simulink library "nmc"  (R2015b)
settings: Solver=ode45  SolverMode=SingleTasking  StartTime=0.0  StopTime=10.0  RelTol=1e-3
undefined symbols (not defined in the file): AFOFS_DIM, alphaFmGas, alphaFmGlu, alphaFmHam, alphaFmSol, alphaFmVas, alphaLceHam, alphaLceHfl, alphaLceTa, alphaLceTa1, Amp, amp_var, c, c_jointstop, CPG, D1G_HAT, DeltaThRef, eref, FmaxGAS, FmaxGLU, FmaxHAM, FmaxHFL, FmaxSOL, FmaxTA, FmaxVAS, freq, freq_var, GainDeltaTheta, GainGAS, GainGLU, GainHAM, GainHAMHFL, GainHFL, GainKneOverExt, GainSOL, GainSOLTA, GainTA, GainVAS, K, K_swing, KneePh23Offset, LceOffsetHAM, LceOffsetHFL, LceOffsetTA, left, LongDelay, loptGAS, loptGLU, loptHAM, loptHFL, loptSOL, loptTA, loptVAS, Lphi230, lslackGAS, lslackGLU, lslackHAM, lslackHFL, lslackSOL, lslackTA ... (+66)
libraries: nmc x94, simulink x29, simulink_extras x17
(part 1 of 5)
settings Model: Creator=efx  LastModifiedBy=efx
settings DataIOCC: SaveFormat=Array
settings OptimizationCC: BlockReduction=off  BooleanDataType=off
settings DebuggingCC: SaveWithParameterizedLinksMsg=none  UnderspecifiedInitializationDetection=Classic  MergeDetectMultiDrivingBlocksExec=none  SignalResolutionControl=TryResolveAllWithWarning  StrictBusMsg=Warning
settings HardwareCC: ProdBitPerPointer=32  ProdLargestAtomicFloat=None  ProdIntDivRoundTo=Undefined  ProdEndianess=Unspecified  ProdWordSize=32  ProdHWDeviceType=32-bit Generic  TargetUnknown=on
settings GRTTargetCC: GeneratePreprocessorConditionals=Disable all
settings ConfigComp: CovModelRefEnable=Off  CovSFcnEnable=off

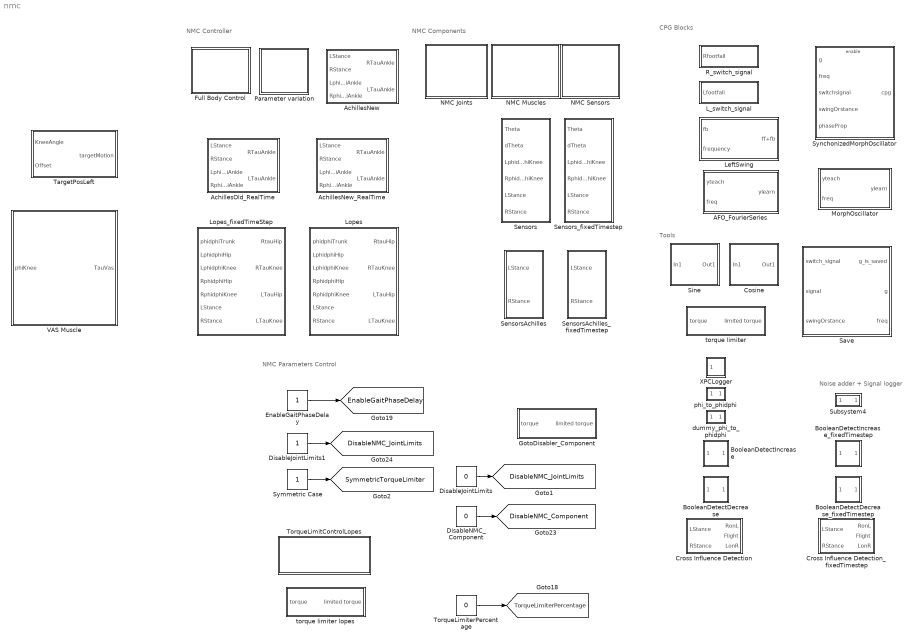
== system nmc ==
  note: Noise adder + Signal logger
  note: NMC Components
  note: Tools
  note: CPG Blocks
  note: NMC Controller
  note: NMC Parameters Control
  AFO_FourierSeries : Subsystem
  AchillesNew : Subsystem
  AchillesNew_RealTime : Subsystem
  AchillesOld_RealTime : Subsystem
  BooleanDetectDecrease : Subsystem
  BooleanDetectDecrease_fixedTimestep : Subsystem
  BooleanDetectIncrease : Subsystem
  BooleanDetectIncrease_fixedTimestep : Subsystem
  Cosine : Subsystem
  Cross Influence Detection : Subsystem
  Cross Influence Detection_fixedTimestep : Subsystem
  DisableJointLimits : Constant  Value=0
  DisableJointLimits1 : Constant
  DisableNMC_Component : Constant  Value=0
  EnableGaitPhaseDelay : Constant
  Full Body Control : Subsystem
  GotoDisabler_Component : Subsystem  mask{GotoTag=DisableNMC_Component}
      mask prompts: GotoTag "Simulink:blkprm_prompts:FromGotoTag"
      mask TypeOptions GotoTag: From/GotoTag
  L_switch_signal : Subsystem
  LeftSwing : Subsystem  InitFcn=CPG.initCurrent();  StopFcn=CPG.saveCurrent();  mask{SaveName=NominalShape1}
      mask prompts: SaveName "Signal nominal shape name"
      mask init:
      | evalin('base','CPG.initCPG();');
      settings: CopyFcn=CPG.initCPG_automaticName();
  Lopes : Subsystem
  Lopes_fixedTimeStep : Subsystem
  MorphOscillator : Subsystem
  NMC Joints : Subsystem
  NMC Muscles : Subsystem
  NMC Sensors : Subsystem
  Parameter variation : Subsystem
  R_switch_signal : Subsystem
  Save : Subsystem
  Sensors : Subsystem
  SensorsAchilles : Subsystem
  SensorsAchilles_fixedTimestep : Subsystem
  Sensors_fixedTimestep : Subsystem
  Sine : Subsystem
  Subsystem4 : Subsystem  mask{GotoTag=LEFT_GLU_FORCE, GotoTag2=LEFT_GLU_FORCE_LOG, GotoTag3=LEFT_GLU_FORCE_NOISE_LOG}
      mask prompts: GotoTag "noise input goto"; GotoTag2 "Goto Logger name"; GotoTag3 "Simulink:blkprm_prompts:GotoTag"
      mask TypeOptions GotoTag: From2/GotoTag
      mask TypeOptions GotoTag2: Goto/GotoTag
      mask TypeOptions GotoTag3: Goto1/GotoTag
  Symmetric Case : Constant
  SynchonizedMorphOscillator : Subsystem
  TargetPosLeft : Subsystem
  TorqueLimitControlLopes : Subsystem
  TorqueLimiterPercentage : Constant  Value=0
  VAS Muscle : Subsystem
  XPCLogger : Subsystem
  dummy_phi_to_phidphi : Subsystem
  phi_to_phidphi : Subsystem
  torque limiter : Subsystem  mask{GotoTag=TorqueLimiterPercentage}
      mask prompts: GotoTag "Simulink:blkprm_prompts:FromGotoTag"
      mask TypeOptions GotoTag: From/GotoTag
  torque limiter lopes : Subsystem  mask{TorqueLimiterPercentage=TorqueLimiterPercentage, EnableTorqueLimiter=EnableTorqueLimiter}
      mask prompts: TorqueLimiterPercentage "Simulink:blkprm_prompts:FromGotoTag"; EnableTorqueLimiter "Simulink:blkprm_prompts:FromGotoTag"
      mask TypeOptions TorqueLimiterPercentage: From/GotoTag
      mask TypeOptions EnableTorqueLimiter: From1/GotoTag
  tag scope: DisableNMC_Component=global, DisableNMC_JointLimits=global, EnableGaitPhaseDelay=global, SymmetricTorqueLimiter=global, TorqueLimiterPercentage=global
  wires:
  TorqueLimiterPercentage/1 -> [TorqueLimiterPercentage]
  DisableNMC_Component/1 -> [DisableNMC_Component]
  DisableJointLimits/1 -> [DisableNMC_JointLimits]
  DisableJointLimits1/1 -> [DisableNMC_JointLimits]
  Symmetric Case/1 -> [SymmetricTorqueLimiter]
  EnableGaitPhaseDelay/1 -> [EnableGaitPhaseDelay]

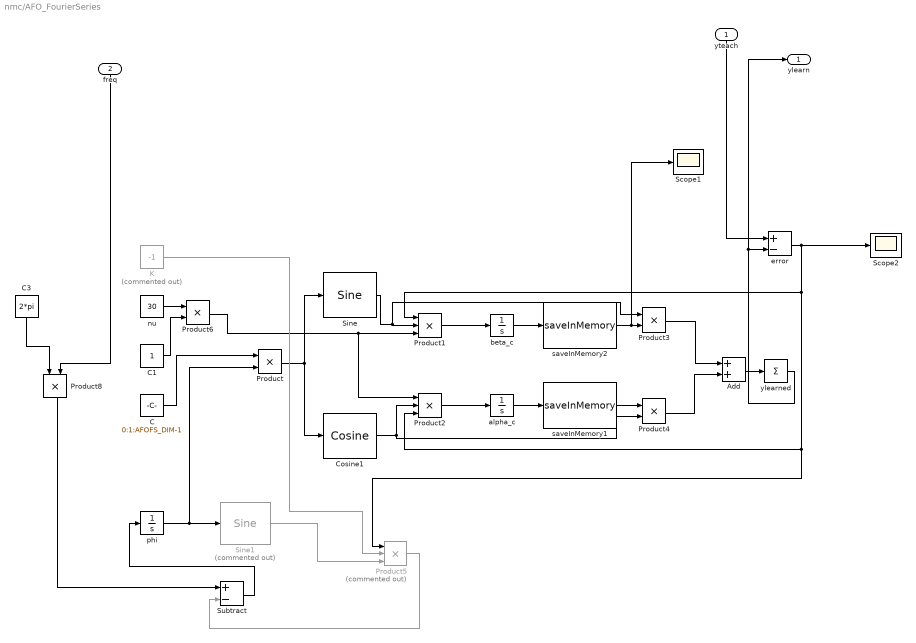
== system nmc/AFO_FourierSeries ==
  yteach : Inport
  freq : Inport  Port=2
  Add : Sum
  C : Constant  Value=0:1:AFOFS_DIM-1
  C1 : Constant
  C3 : Constant  Value=2*pi
  Cosine1 : nmc/Cosine
  K : Constant  Commented=on  Value=-1
  Product{,3..4,6,8} (5 alike) : Product
  Product1 : Product  Inputs=3
  Product2 : Product  Inputs=3
  Product5 : Product  Commented=on  Inputs=3
  Scope1 : Scope
  Scope2 : Scope
  Sine : nmc/Sine
  Sine1 : simulink/Lookup Tables/Sine  Commented=on  Formula=sin(2*pi*u)  NumDataPoints=(2^5)+1  OutputWordLength=16  InternalRulePriority=Speed
  Subtract : Sum  Inputs=+-
  alpha_c : Integrator
  beta_c : Integrator
  error : Sum  Inputs=+-
  nu : Constant  Value=30
  phi : Integrator
  saveInMemory1 : nmc/saveInMemory
  saveInMemory2 : nmc/saveInMemory
  ylearned : Sum  Inputs=+
  ylearn : Outport
  wires:
  saveInMemory2/1 -> Product3/2, Scope1/1
  saveInMemory1/1 -> Product4/1
  yteach/1 -> error/1
  Subtract/1 -> phi/1
  Product6/1 -> Product2/1, Product1/3
  Sine1/1 -> Product5/3
  nu/1 -> Product6/1
  C1/1 -> Product6/2
  Product/1 -> Cosine1/1, Sine/1
  Product1/1 -> beta_c/1
  Product2/1 -> alpha_c/1
  beta_c/1 -> saveInMemory2/1
  alpha_c/1 -> saveInMemory1/1
  Product3/1 -> Add/1
  Product4/1 -> Add/2
  Add/1 -> ylearned/1
  ylearned/1 -> ylearn/1, error/2
  K/1 -> Product5/2
  error/1 -> Product1/1, Product2/3, Product5/1, Scope2/1
  Product5/1 -> Subtract/2
  Product8/1 -> Subtract/1
  phi/1 -> Sine1/1, Product/2
  C/1 -> Product/1
  Sine/1 -> Product1/2, Product3/1
  Cosine1/1 -> Product2/2, Product4/2
  freq/1 -> Product8/2
  C3/1 -> Product8/1

== system nmc/AchillesNew ==
  LStance : Inport
  RStance : Inport  Port=2
  LphidphiAnkle : Inport  Port=3
  RphidphiAnkle : Inport  Port=4
  Left Side : Subsystem
  Right Side : Subsystem
  SensorsAchilles : nmc/SensorsAchilles
  RTauAnkle : Outport
  LTauAnkle : Outport  Port=2
  wires:
  [RTauAnkle] -> RTauAnkle/1
  [LTauAnkle] -> LTauAnkle/1
  Left Side/1(LTauAnkle) -> [LTauAnkle]
  Right Side/1(RTauAnkle) -> [RTauAnkle]
  [RphidphiAnkle] -> Right Side/1(RphidphiAnkle)
  [LphidphiAnkle] -> Left Side/1(LphidphiAnkle)
  RphidphiAnkle/1 -> [RphidphiAnkle]
  LphidphiAnkle/1 -> [LphidphiAnkle]
  [LStance] -> SensorsAchilles/1
  [RStance] -> SensorsAchilles/2
  LStance/1 -> [LStance]
  RStance/1 -> [RStance]

== system nmc/AchillesNew_RealTime ==
  LStance : Inport
  RStance : Inport  Port=2
  LphidphiAnkle : Inport  Port=3
  RphidphiAnkle : Inport  Port=4
  Left Side : Subsystem
  Right Side : Subsystem
  SensorsAchilles_fixedTimestep : nmc/SensorsAchilles_fixedTimestep
  RTauAnkle : Outport
  LTauAnkle : Outport  Port=2
  wires:
  RStance/1 -> [RStance]
  LStance/1 -> [LStance]
  [RStance] -> SensorsAchilles_fixedTimestep/2
  [LStance] -> SensorsAchilles_fixedTimestep/1
  LphidphiAnkle/1 -> [LphidphiAnkle]
  RphidphiAnkle/1 -> [RphidphiAnkle]
  [LphidphiAnkle] -> Left Side/1(LphidphiAnkle)
  [RphidphiAnkle] -> Right Side/1(RphidphiAnkle)
  Right Side/1(RTauAnkle) -> [RTauAnkle]
  Left Side/1(LTauAnkle) -> [LTauAnkle]
  [LTauAnkle] -> LTauAnkle/1
  [RTauAnkle] -> RTauAnkle/1

== system nmc/AchillesOld_RealTime ==
  LStance : Inport
  RStance : Inport  Port=2
  LphidphiAnkle : Inport  Port=3
  RphidphiAnkle : Inport  Port=4
  Achilles : Subsystem
  SensorsAchilles_fixedTimestep : nmc/SensorsAchilles_fixedTimestep
  RTauAnkle : Outport
  LTauAnkle : Outport  Port=2
  wires:
  [RTauAnkle] -> RTauAnkle/1
  [LTauAnkle] -> LTauAnkle/1
  Achilles/1(Torque) -> [LTauAnkle]
  [LphidphiAnkle] -> Achilles/1(AngleLeft)
  RphidphiAnkle/1 -> [RphidphiAnkle]
  LphidphiAnkle/1 -> [LphidphiAnkle]
  [LStance] -> SensorsAchilles_fixedTimestep/1
  [RStance] -> SensorsAchilles_fixedTimestep/2
  LStance/1 -> [LStance]
  RStance/1 -> [RStance]
  [RphidphiAnkle] -> Achilles/3(AngleRight)
  [LstanceOut] -> Achilles/2(IsStanceLeft)
  [RstanceOut] -> Achilles/4(IsStanceRight)
  Achilles/2(Torque1) -> [RTauAnkle]

== system nmc/BooleanDetectDecrease ==
  In1 : Inport
  Compare To Constant : simulink/Logic and Bit Operations/Compare To Constant  relop===  const=-1  OutDataTypeStr=boolean
  Data Type Conversion : DataTypeConversion
  Memory1 : Memory
  Sum : Sum  Inputs=|+-
  Out1 : Outport
  wires:
  Data Type Conversion/1 -> Out1/1
  In1/1 -> Memory1/1, Sum/1
  Sum/1 -> Compare To Constant/1
  Compare To Constant/1 -> Data Type Conversion/1
  Memory1/1 -> Sum/2

== system nmc/BooleanDetectDecrease_fixedTimestep ==
  In1 : Inport
  Data Type Conversion : DataTypeConversion
  Detect Decrease : simulink/Logic and Bit Operations/Detect Decrease  vinit=0.0  InputProcessing=Inherited  OutDataTypeStr=boolean
  Out1 : Outport
  wires:
  In1/1 -> Detect Decrease/1
  Data Type Conversion/1 -> Out1/1
  Detect Decrease/1 -> Data Type Conversion/1

== system nmc/BooleanDetectIncrease ==
  In1 : Inport
  Compare To Constant : simulink/Logic and Bit Operations/Compare To Constant  relop===  const=1  OutDataTypeStr=boolean
  Data Type Conversion : DataTypeConversion
  Memory1 : Memory
  Sum : Sum  Inputs=|+-
  Out1 : Outport
  wires:
  Data Type Conversion/1 -> Out1/1
  In1/1 -> Memory1/1, Sum/1
  Sum/1 -> Compare To Constant/1
  Compare To Constant/1 -> Data Type Conversion/1
  Memory1/1 -> Sum/2

== system nmc/BooleanDetectIncrease_fixedTimestep ==
  In1 : Inport
  Data Type Conversion : DataTypeConversion
  Detect Increase : simulink/Logic and Bit Operations/Detect Increase  vinit=0  InputProcessing=Inherited  OutDataTypeStr=boolean
  Out1 : Outport
  wires:
  Detect Increase/1 -> Data Type Conversion/1
  In1/1 -> Detect Increase/1
  Data Type Conversion/1 -> Out1/1

== system nmc/Cosine ==
  In1 : Inport
  MATLAB Function1 : MATLAB Function  TreatAsAtomicUnit=on
  Out1 : Outport
  wires:
  In1/1 -> MATLAB Function1/1(t)
  MATLAB Function1/1(y) -> Out1/1

== system nmc/Cross Influence Detection ==
  note: Double Support Cross Influences
  note: right leg is leading
  note: left leg is leading
  LStance : Inport  OutDataTypeStr=double
  RStance : Inport  Port=2  OutDataTypeStr=double
  BooleanDetectDecrease : nmc/BooleanDetectDecrease
  BooleanDetectIncrease : nmc/BooleanDetectIncrease
  BooleanDetectIncrease1 : nmc/BooleanDetectIncrease
  Data Type Conversion1 : DataTypeConversion
  Data Type Conversion2 : DataTypeConversion
  Data Type Conversion3 : DataTypeConversion
  Double Support? : Logic  AllPortsSameDT=off
  Double Support?1 : Logic  AllPortsSameDT=off
  Double Support?4 : Logic  AllPortsSameDT=off
  Flight? : Logic  Operator=NOR  AllPortsSameDT=off
  Memory : Memory
  Memory3 : Memory
  S-R Flip-Flop : simulink_extras/Flip Flops/S-R Flip-Flop  initial_condition=0
  S-R Flip-Flop1 : simulink_extras/Flip Flops/S-R Flip-Flop  initial_condition=0
  Terminator1 : Terminator
  Terminator2 : Terminator
  RonL : Outport  OutDataTypeStr=double
  Flight : Outport  Port=2  OutDataTypeStr=double
  LonR : Outport  Port=3  OutDataTypeStr=double
  wires:
  Double Support?1/1 -> S-R Flip-Flop1/1
  BooleanDetectIncrease1/1 -> Double Support?1/2
  S-R Flip-Flop/2 -> Terminator1/1
  S-R Flip-Flop1/2 -> Terminator2/1
  Memory/1 -> BooleanDetectIncrease1/1
  LStance/1 -> Memory3/1, Double Support?/1, Flight?/1
  BooleanDetectIncrease/1 -> Double Support?4/1
  Double Support?4/1 -> S-R Flip-Flop/1
  Memory3/1 -> BooleanDetectIncrease/1
  RStance/1 -> Memory/1, Double Support?/2, Flight?/2
  Double Support?/1 -> BooleanDetectDecrease/1, Double Support?1/1, Double Support?4/2
  S-R Flip-Flop/1 -> Data Type Conversion2/1
  Flight?/1 -> Data Type Conversion1/1
  S-R Flip-Flop1/1 -> Data Type Conversion3/1
  Data Type Conversion1/1 -> Flight/1
  Data Type Conversion2/1 -> LonR/1
  Data Type Conversion3/1 -> RonL/1
  BooleanDetectDecrease/1 -> S-R Flip-Flop/2, S-R Flip-Flop1/2

== system nmc/Cross Influence Detection_fixedTimestep ==
  note: left leg is leading
  note: right leg is leading
  note: Double Support Cross Influences
  LStance : Inport  OutDataTypeStr=double
  RStance : Inport  Port=2  OutDataTypeStr=double
  BooleanDetectDecrease_fixedTimestep : nmc/BooleanDetectDecrease_fixedTimestep
  BooleanDetectIncrease_fixedTimestep : nmc/BooleanDetectIncrease_fixedTimestep
  BooleanDetectIncrease_fixedTimestep1 : nmc/BooleanDetectIncrease_fixedTimestep
  Data Type Conversion1 : DataTypeConversion
  Data Type Conversion2 : DataTypeConversion
  Data Type Conversion3 : DataTypeConversion
  Double Support? : Logic  AllPortsSameDT=off
  Double Support?1 : Logic  AllPortsSameDT=off
  Double Support?4 : Logic  AllPortsSameDT=off
  Flight? : Logic  Operator=NOR  AllPortsSameDT=off
  Memory : Memory
  Memory3 : Memory
  S-R Flip-Flop : simulink_extras/Flip Flops/S-R Flip-Flop  initial_condition=0
  S-R Flip-Flop1 : simulink_extras/Flip Flops/S-R Flip-Flop  initial_condition=0
  Terminator1 : Terminator
  Terminator2 : Terminator
  RonL : Outport  OutDataTypeStr=double
  Flight : Outport  Port=2  OutDataTypeStr=double
  LonR : Outport  Port=3  OutDataTypeStr=double
  wires:
  BooleanDetectDecrease_fixedTimestep/1 -> S-R Flip-Flop1/2, S-R Flip-Flop/2
  Data Type Conversion3/1 -> RonL/1
  Data Type Conversion2/1 -> LonR/1
  Data Type Conversion1/1 -> Flight/1
  S-R Flip-Flop1/1 -> Data Type Conversion3/1
  Flight?/1 -> Data Type Conversion1/1
  S-R Flip-Flop/1 -> Data Type Conversion2/1
  Double Support?/1 -> Double Support?4/2, BooleanDetectDecrease_fixedTimestep/1, Double Support?1/1
  RStance/1 -> Flight?/2, Double Support?/2, Memory/1
  Memory3/1 -> BooleanDetectIncrease_fixedTimestep/1
  Double Support?4/1 -> S-R Flip-Flop/1
  BooleanDetectIncrease_fixedTimestep/1 -> Double Support?4/1
  LStance/1 -> Flight?/1, Double Support?/1, Memory3/1
  Memory/1 -> BooleanDetectIncrease_fixedTimestep1/1
  S-R Flip-Flop1/2 -> Terminator2/1
  S-R Flip-Flop/2 -> Terminator1/1
  BooleanDetectIncrease_fixedTimestep1/1 -> Double Support?1/2
  Double Support?1/1 -> S-R Flip-Flop1/1

== system nmc/Full Body Control ==
  Left Side : Subsystem
  Right Side : Subsystem
  Sensors : Subsystem

== system nmc/GotoDisabler_Component ==
  torque : Inport
  Product : Product
  limited torque : Outport
  wires:
  [DisableNMC_Component] -> Product/1
  Product/1 -> limited torque/1
  torque/1 -> Product/2

== system nmc/L_switch_signal ==
  Lfootfall : Inport
  Memory : Memory
  Subtract : Sum  Inputs=+-
  tag scope: CPG_leftSwitchSignal=global
  wires:
  Subtract/1 -> [CPG_leftSwitchSignal]
  Lfootfall/1 -> Memory/1, Subtract/1
  Memory/1 -> Subtract/2

== system nmc/LeftSwing ==
  fb : Inport
  frequency : Inport  Port=2
  AlreadySavedInWorkspace : Constant  Value=CPG.Signals.NominalShape1.Enabled
  CPG : Subsystem
  ChooseOutput : Switch  Criteria=u2 > Threshold  Threshold=0.5
  GenerateAndSaveNominalShape : Subsystem
  LeftOrRight : Subsystem
  Logical Operator : Logic  Operator=NOT  Inputs=1  AllPortsSameDT=off  OutDataTypeStr=boolean
  leftOrright : Constant  Value=left
  swingOrstance : Constant  Value=swing
  ff+fb : Outport
  wires:
  LeftOrRight/1(switch_signal) -> GenerateAndSaveNominalShape/1(switch_signal)
  leftOrright/1 -> LeftOrRight/1(side)
  ChooseOutput/1 -> ff+fb/1
  frequency/1 -> CPG/1(freq)
  CPG/1(y) -> ChooseOutput/1
  Logical Operator/1 -> GenerateAndSaveNominalShape/Enable
  swingOrstance/1 -> GenerateAndSaveNominalShape/3(swingOrstance)
  fb/1 -> ChooseOutput/3, GenerateAndSaveNominalShape/2(signal)
  AlreadySavedInWorkspace/1 -> CPG/Enable, ChooseOutput/2, Logical Operator/1

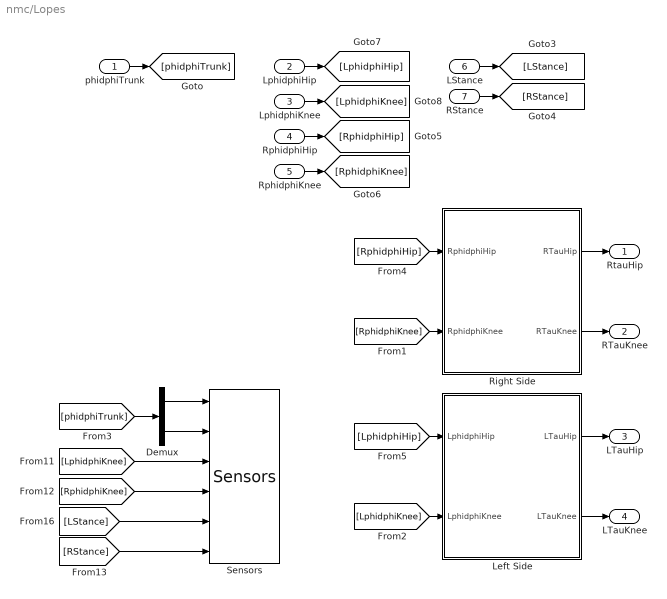
== system nmc/Lopes ==
  phidphiTrunk : Inport
  LphidphiHip : Inport  Port=2
  LphidphiKnee : Inport  Port=3
  RphidphiHip : Inport  Port=4
  RphidphiKnee : Inport  Port=5
  LStance : Inport  Port=6
  RStance : Inport  Port=7
  Demux : Demux  Outputs=2
  Left Side : Subsystem
  Right Side : Subsystem
  Sensors : nmc/Sensors
  RtauHip : Outport
  RTauKnee : Outport  Port=2
  LTauHip : Outport  Port=3
  LTauKnee : Outport  Port=4
  wires:
  RphidphiKnee/1 -> [RphidphiKnee]
  LphidphiHip/1 -> [LphidphiHip]
  LphidphiKnee/1 -> [LphidphiKnee]
  RphidphiHip/1 -> [RphidphiHip]
  RStance/1 -> [RStance]
  LStance/1 -> [LStance]
  phidphiTrunk/1 -> [phidphiTrunk]
  Left Side/2(LTauKnee) -> LTauKnee/1
  Left Side/1(LTauHip) -> LTauHip/1
  Right Side/2(RTauKnee) -> RTauKnee/1
  Right Side/1(RTauHip) -> RtauHip/1
  [LphidphiHip] -> Left Side/1(LphidphiHip)
  [RphidphiHip] -> Right Side/1(RphidphiHip)
  Demux/2 -> Sensors/2
  Demux/1 -> Sensors/1
  [phidphiTrunk] -> Demux/1
  [LphidphiKnee] -> Left Side/2(LphidphiKnee)
  [RphidphiKnee] -> Right Side/2(RphidphiKnee)
  [RStance] -> Sensors/6
  [LStance] -> Sensors/5
  [RphidphiKnee] -> Sensors/4
  [LphidphiKnee] -> Sensors/3

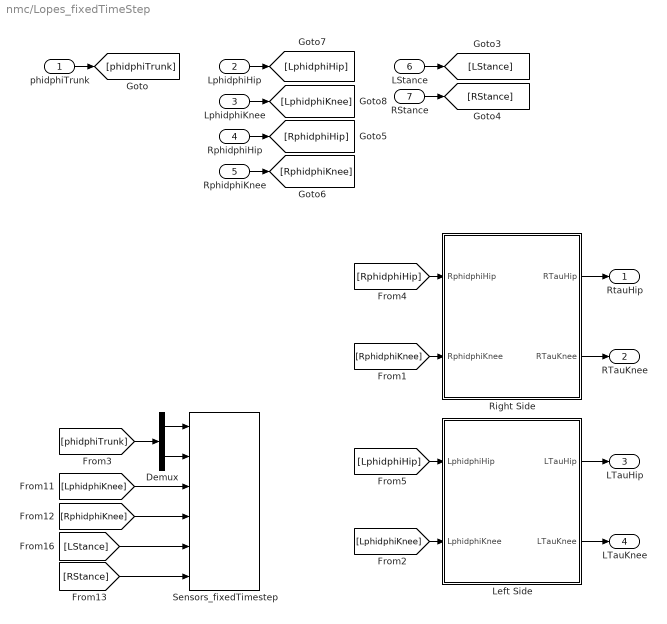
== system nmc/Lopes_fixedTimeStep ==
  phidphiTrunk : Inport
  LphidphiHip : Inport  Port=2
  LphidphiKnee : Inport  Port=3
  RphidphiHip : Inport  Port=4
  RphidphiKnee : Inport  Port=5
  LStance : Inport  Port=6
  RStance : Inport  Port=7
  Demux : Demux  Outputs=2
  Left Side : Subsystem
  Right Side : Subsystem
  Sensors_fixedTimestep : nmc/Sensors_fixedTimestep
  RtauHip : Outport
  RTauKnee : Outport  Port=2
  LTauHip : Outport  Port=3
  LTauKnee : Outport  Port=4
  wires:
  [LphidphiKnee] -> Sensors_fixedTimestep/3
  [RphidphiKnee] -> Sensors_fixedTimestep/4
  [LStance] -> Sensors_fixedTimestep/5
  [RStance] -> Sensors_fixedTimestep/6
  [RphidphiKnee] -> Right Side/2(RphidphiKnee)
  [LphidphiKnee] -> Left Side/2(LphidphiKnee)
  [phidphiTrunk] -> Demux/1
  Demux/1 -> Sensors_fixedTimestep/1
  Demux/2 -> Sensors_fixedTimestep/2
  [RphidphiHip] -> Right Side/1(RphidphiHip)
  [LphidphiHip] -> Left Side/1(LphidphiHip)
  Right Side/1(RTauHip) -> RtauHip/1
  Right Side/2(RTauKnee) -> RTauKnee/1
  Left Side/1(LTauHip) -> LTauHip/1
  Left Side/2(LTauKnee) -> LTauKnee/1
  phidphiTrunk/1 -> [phidphiTrunk]
  LStance/1 -> [LStance]
  RStance/1 -> [RStance]
  RphidphiHip/1 -> [RphidphiHip]
  LphidphiKnee/1 -> [LphidphiKnee]
  LphidphiHip/1 -> [LphidphiHip]
  RphidphiKnee/1 -> [RphidphiKnee]

== system nmc/MorphOscillator ==
  yteach : Inport
  freq : Inport  Port=2
  Digital Clock : DigitalClock  SampleTime=0.001
  MATLAB Function : MATLAB Function  TreatAsAtomicUnit=on
  ylearn : Outport  SampleTime=0.001
  wires:
  freq/1 -> MATLAB Function/2(freq)
  yteach/1 -> MATLAB Function/1(g)
  Digital Clock/1 -> MATLAB Function/3(t)
  MATLAB Function/1(y) -> ylearn/1

== system nmc/NMC Joints ==
  AnkleJoint : Subsystem
  HipJoint : Subsystem
  KneeJoint : Subsystem

== system nmc/NMC Muscles ==
  note: NMC Muscles
  GAS Muscle : Subsystem  mask{VariableName=StimGAS, GASVM=GASL_VM}
      mask prompts: VariableName "Simulink:blkprm_prompts:ToWksVarName"; GASVM "Simulink:blkprm_prompts:GotoTag"
      mask TypeOptions VariableName: StimGAS/VariableName
      mask TypeOptions GASVM: GAS Actuation / GAS_VM/GotoTag
  GLU Muscle : Subsystem  mask{StimGluSide=StimGLUR, GotoTag=GLUR_VM}
      mask prompts: StimGluSide "Simulink:blkprm_prompts:ToWksVarName"; GotoTag "Simulink:blkprm_prompts:GotoTag"
      mask TypeOptions StimGluSide: StimGLU/VariableName
      mask TypeOptions GotoTag: GLU Actuation/GLU_VM /GotoTag
  "HFL Muscle " : Subsystem  mask{VariableName=StimHFL}
      mask prompts: VariableName "Simulink:blkprm_prompts:ToWksVarName"
      mask TypeOptions VariableName: StimHFL/VariableName
  HFL&HAM Muscles : Subsystem  mask{StimHAMSide=StimHAMR, StimHFLSide=StimHFLR, HAMVM=HAMR_VM, HFLVM=HFLR_VM}
      mask prompts: StimHAMSide "Simulink:blkprm_prompts:ToWksVarName"; StimHFLSide "Simulink:blkprm_prompts:ToWksVarName"; HAMVM "Simulink:blkprm_prompts:GotoTag"; HFLVM "Simulink:blkprm_prompts:GotoTag"
      mask TypeOptions StimHAMSide: StimHAM/VariableName
      mask TypeOptions StimHFLSide: StimHFL/VariableName
      mask TypeOptions HAMVM: HAM Actuation / HAM_VM/GotoTag
      mask TypeOptions HFLVM: HFL Actuation/ HFL_VM/GotoTag
  SOL&TA Muscles : Subsystem  mask{VariableName=StimSOL, VariableNameTA=StimTA, SOLVM=SOLL_VM, TAVM=TAL_VM}
      mask prompts: VariableName "Simulink:blkprm_prompts:ToWksVarName"; VariableNameTA "Simulink:blkprm_prompts:ToWksVarName"; SOLVM "Simulink:blkprm_prompts:GotoTag"; TAVM "Simulink:blkprm_prompts:GotoTag"
      mask TypeOptions VariableName: StimSOL/VariableName
      mask TypeOptions VariableNameTA: StimTA/VariableName
      mask TypeOptions SOLVM: SOL Actuation/SOL_VM/GotoTag
      mask TypeOptions TAVM: TA Actuation/TA_VM/GotoTag
  VAS Muscle : Subsystem  mask{VariableName=StimVASR, VASVM=VASR_VM}
      mask prompts: VariableName "Simulink:blkprm_prompts:ToWksVarName"; VASVM "Simulink:blkprm_prompts:GotoTag"
      mask TypeOptions VariableName: StimVAS/VariableName
      mask TypeOptions VASVM: VAS Actuation / VAS_VM/GotoTag

== system nmc/NMC Sensors ==
  FootSensor : Subsystem
  FootSensorSimple : Subsystem
  FootSensor_fixedTimestep : Subsystem
  GeyerUpperBodyOrientation : Subsystem
  KneeSensor : Subsystem
  ThightSensor : Subsystem
  ThightSensorSimulator : Subsystem
  UpperBodyOrientation : Subsystem

== system nmc/Parameter variation ==
  Alpha variation : Subsystem
  Amplitude Variation : Subsystem
  Freq variation : Subsystem

== system nmc/R_switch_signal ==
  Rfootfall : Inport
  Memory : Memory
  Subtract : Sum  Inputs=+-
  tag scope: CPG_rightSwitchSignal=global
  wires:
  Rfootfall/1 -> Subtract/1, Memory/1
  Memory/1 -> Subtract/2
  Subtract/1 -> [CPG_rightSwitchSignal]

== system nmc/Save ==
  switch_signal : Inport
  signal : Inport  Port=2
  "swingOrstance " : Inport  Port=3
  N_record : Constant  Value=N_record
  N_start : Constant  Value=N_start
  save : Stateflow chart  TreatAsAtomicUnit=on
  g_is_saved : Outport
  g : Outport  Port=2
  freq : Outport  Port=3
  wires:
  save/3(saved) -> g_is_saved/1
  "swingOrstance "/1 -> save/5(swingOrstance)
  save/1(g) -> g/1
  N_start/1 -> save/2(N_start)
  save/2(freq) -> freq/1
  signal/1 -> save/4(signal)
  N_record/1 -> save/3(N_record)
  switch_signal/1 -> save/1(switch_signal)

== system nmc/Sensors ==
  Theta : Inport
  dTheta : Inport  Port=2
  LphidphiKnee : Inport  Port=3
  RphidphiKnee : Inport  Port=4
  LStance : Inport  Port=5
  RStance : Inport  Port=6
  Body Pitch loop delay : TransportDelay  DelayTime=ShortDelay
  Body Pitch loop delay. : TransportDelay  DelayTime=ShortDelay
  FootSensor : nmc/NMC Sensors/FootSensor
  KneeSensor : nmc/NMC Sensors/KneeSensor
  ThightSensorSimulator : nmc/NMC Sensors/ThightSensorSimulator
  To Workspace : ToWorkspace  VariableName=L_GRF  SaveFormat=Timeseries  SampleTime=-1
  To Workspace1 : ToWorkspace  VariableName=R_GRF  SaveFormat=Timeseries  SampleTime=-1
  tag scope: LKneeStateOut=global, LdxThighOut=global, LonR=global, LstanceOut=global, RKneeStateOut=global, RdxThighOut=global, RonL=global, RstanceOut=global, ThetaDelayed=global, dThetaDelayed=global
  wires:
  LphidphiKnee/1 -> KneeSensor/1
  RphidphiKnee/1 -> KneeSensor/2
  KneeSensor/1 -> [LKneeStateOut]
  KneeSensor/2 -> [RKneeStateOut]
  FootSensor/1 -> [LstanceOut]
  FootSensor/2 -> [RstanceOut]
  FootSensor/3 -> [LonR]
  FootSensor/4 -> [RonL]
  ThightSensorSimulator/1 -> [LdxThighOut]
  ThightSensorSimulator/2 -> [RdxThighOut]
  [rightGRF_vertical] -> To Workspace1/1
  [leftGRF_vertical] -> To Workspace/1
  [LstanceOut] -> ThightSensorSimulator/1
  [RstanceOut] -> ThightSensorSimulator/2
  RStance/1 -> FootSensor/2
  LStance/1 -> FootSensor/1
  Theta/1 -> Body Pitch loop delay./1
  dTheta/1 -> Body Pitch loop delay/1
  Body Pitch loop delay./1 -> [ThetaDelayed]
  Body Pitch loop delay/1 -> [dThetaDelayed]

== system nmc/SensorsAchilles ==
  LStance : Inport
  RStance : Inport  Port=2
  FootSensor : nmc/NMC Sensors/FootSensor
  tag scope: LonR=global, LstanceOut=global, RonL=global, RstanceOut=global
  wires:
  LStance/1 -> FootSensor/1
  RStance/1 -> FootSensor/2
  FootSensor/4 -> [RonL]
  FootSensor/3 -> [LonR]
  FootSensor/2 -> [RstanceOut]
  FootSensor/1 -> [LstanceOut]

== system nmc/SensorsAchilles_fixedTimestep ==
  LStance : Inport
  RStance : Inport  Port=2
  FootSensor_fixedTimestep : nmc/NMC Sensors/FootSensor_fixedTimestep
  tag scope: LonR=global, LstanceOut=global, RonL=global, RstanceOut=global
  wires:
  FootSensor_fixedTimestep/1 -> [LstanceOut]
  FootSensor_fixedTimestep/2 -> [RstanceOut]
  FootSensor_fixedTimestep/3 -> [LonR]
  FootSensor_fixedTimestep/4 -> [RonL]
  RStance/1 -> FootSensor_fixedTimestep/2
  LStance/1 -> FootSensor_fixedTimestep/1

== system nmc/Sensors_fixedTimestep ==
  Theta : Inport
  dTheta : Inport  Port=2
  LphidphiKnee : Inport  Port=3
  RphidphiKnee : Inport  Port=4
  LStance : Inport  Port=5
  RStance : Inport  Port=6
  Body Pitch loop delay : TransportDelay  DelayTime=ShortDelay
  Body Pitch loop delay. : TransportDelay  DelayTime=ShortDelay
  FootSensor_fixedTimestep : nmc/NMC Sensors/FootSensor_fixedTimestep
  KneeSensor : nmc/NMC Sensors/KneeSensor
  ThightSensorSimulator : nmc/NMC Sensors/ThightSensorSimulator
  To Workspace : ToWorkspace  VariableName=L_GRF  SaveFormat=Timeseries  SampleTime=-1
  To Workspace1 : ToWorkspace  VariableName=R_GRF  SaveFormat=Timeseries  SampleTime=-1
  tag scope: LKneeStateOut=global, LdxThighOut=global, LonR=global, LstanceOut=global, RKneeStateOut=global, RdxThighOut=global, RonL=global, RstanceOut=global, ThetaDelayed=global, dThetaDelayed=global
  wires:
  Body Pitch loop delay/1 -> [dThetaDelayed]
  Body Pitch loop delay./1 -> [ThetaDelayed]
  dTheta/1 -> Body Pitch loop delay/1
  Theta/1 -> Body Pitch loop delay./1
  LStance/1 -> FootSensor_fixedTimestep/1
  RStance/1 -> FootSensor_fixedTimestep/2
  [RstanceOut] -> ThightSensorSimulator/2
  [LstanceOut] -> ThightSensorSimulator/1
  [leftGRF_vertical] -> To Workspace/1
  [rightGRF_vertical] -> To Workspace1/1
  ThightSensorSimulator/2 -> [RdxThighOut]
  ThightSensorSimulator/1 -> [LdxThighOut]
  FootSensor_fixedTimestep/4 -> [RonL]
  FootSensor_fixedTimestep/3 -> [LonR]
  FootSensor_fixedTimestep/2 -> [RstanceOut]
  FootSensor_fixedTimestep/1 -> [LstanceOut]
  KneeSensor/2 -> [RKneeStateOut]
  KneeSensor/1 -> [LKneeStateOut]
  RphidphiKnee/1 -> KneeSensor/2
  LphidphiKnee/1 -> KneeSensor/1

== system nmc/Sine ==
  In1 : Inport
  MATLAB Function1 : MATLAB Function  TreatAsAtomicUnit=on
  Out1 : Outport
  wires:
  MATLAB Function1/1(y) -> Out1/1
  In1/1 -> MATLAB Function1/1(t)

== system nmc/Subsystem4 ==
  In1 : Inport
  Constant : Constant  Value=0
  Sum : Sum  Inputs=|++
  Switch : Switch  Criteria=u2 > Threshold
  Out1 : Outport
  tag scope: LEFT_GLU_FORCE_LOG=global, LEFT_GLU_FORCE_NOISE_LOG=global
  wires:
  In1/1 -> Sum/2, [LEFT_GLU_FORCE_LOG]
  [LEFT_GLU_FORCE] -> Sum/1
  Sum/1 -> Switch/1, Switch/2
  Constant/1 -> Switch/3
  Switch/1 -> [LEFT_GLU_FORCE_NOISE_LOG], Out1/1

== system nmc/SynchonizedMorphOscillator ==
  g : Inport
  freq : Inport  Port=2
  switchsignal : Inport  Port=3
  swingOrstance : Inport  Port=4
  phaseProp : Inport  Port=5
  Enable : EnablePort
  ConstantCPG : Subsystem
  Logical Operator : Logic  Operator=NOT  AllPortsSameDT=off  OutDataTypeStr=boolean
  Memory : Memory
  Memory1 : Memory
  Memory2 : Memory
  MorphingOscillator : Subsystem
  State Transition Table : State Transition Table  TreatAsAtomicUnit=on
  Switch : Switch  Criteria=u2 > Threshold
  enable cpg : Subsystem
  cpg : Outport
  wires:
  MorphingOscillator/2(tetha_out) -> Memory/1
  swingOrstance/1 -> MorphingOscillator/4(swingOrstance), State Transition Table/2(swingOrstance)
  freq/1 -> MorphingOscillator/2(freq)
  g/1 -> MorphingOscillator/1(g)
  State Transition Table/1(actif) -> Logical Operator/1, enable cpg/Enable, Switch/2
  State Transition Table/2(cpg_cnst) -> ConstantCPG/1(cpg_cnst_value)
  Logical Operator/1 -> ConstantCPG/Enable
  ConstantCPG/1(cpg_value) -> Switch/3
  Switch/1 -> cpg/1
  switchsignal/1 -> MorphingOscillator/3(switchsignal), Memory2/1
  Memory1/1 -> State Transition Table/3(cpg)
  Memory/1 -> State Transition Table/4(tetha)
  MorphingOscillator/1(cpg) -> Memory1/1, enable cpg/1(cpg_on)
  enable cpg/1(cpg) -> Switch/1
  Memory2/1 -> State Transition Table/1(switchsignal)
  phaseProp/1 -> State Transition Table/5(phaseProp)

== system nmc/TargetPosLeft ==
  KneeAngle : Inport
  Offset : Inport  Port=2
  Add : Sum  Inputs=-+
  Add1 : Sum
  Constant : Constant  Value=0
  Constant1 : Constant  Value=pi
  Demux4 : Demux  Outputs=2
  Gain : Gain  Gain=0.5
  Memory : Memory  X0=Lphi230
  Mux1 : Mux  Inputs=3
  Terminator : Terminator
  targetMotion : Outport
  wires:
  KneeAngle/1 -> Memory/1
  Mux1/1 -> targetMotion/1
  Demux4/2 -> Terminator/1
  Constant/1 -> Mux1/3, Mux1/2
  Add/1 -> Gain/1
  Demux4/1 -> Add/2
  Constant1/1 -> Add/1
  Gain/1 -> Add1/2
  Add1/1 -> Mux1/1
  Offset/1 -> Add1/1
  Memory/1 -> Demux4/1

== system nmc/TorqueLimitControlLopes ==
  Constant6 : Constant
  Subtract : Sum  Inputs=-+
  tag scope: EnableAssymmetricTorqueLimiter=global, EnableSymmetricTorqueLimiter=global
  wires:
  [SymmetricTorqueLimiter] -> Subtract/1, [EnableSymmetricTorqueLimiter]
  Subtract/1 -> [EnableAssymmetricTorqueLimiter]
  Constant6/1 -> Subtract/2

== system nmc/VAS Muscle ==
  note: VAS Control
  note: VAS Muscle
  note: VAS Control
  phiKnee : Inport
  "ANMC STIM " : Concatenate  NumInputs=1
  Gain : Gain  Gain=GainVAS
  LOG_TauVas : Concatenate  NumInputs=1
  Saturation17 : Saturate  UpperLimit=1  LowerLimit=0.01  ZeroCross=off
  Stimulation Bias : Constant  Value=PreStimVAS
  Sum2 : Sum  Inputs=|++  SaturateOnIntegerOverflow=on  InputSameDT=on  OutDataTypeStr=Inherit: Same as first input
  "VAS Actuation " : Subsystem
  TauVas : Outport
  wires:
  LOG_TauVas/1 -> TauVas/1
  "ANMC STIM "/1 -> "VAS Actuation "/2(StimVas)
  "VAS Actuation "/1(TauVas) -> LOG_TauVas/1
  phiKnee/1 -> "VAS Actuation "/1(phiKnee)
  "VAS Actuation "/2(FmVas) -> Gain/1
  Gain/1 -> Sum2/2
  Stimulation Bias/1 -> Sum2/1
  Sum2/1 -> Saturation17/1
  Saturation17/1 -> "ANMC STIM "/1

== system nmc/XPCLogger ==
  In1 : Inport
  Terminator5 : Terminator
  wires:
  In1/1 -> Terminator5/1

== system nmc/dummy_phi_to_phidphi ==
  phi : Inport
  Constant : Constant  Value=0
  Mux : Mux  Inputs=2
  phi_dummydphi : Outport
  wires:
  Mux/1 -> phi_dummydphi/1
  phi/1 -> Mux/2
  Constant/1 -> Mux/1

== system nmc/phi_to_phidphi ==
  phi : Inport
  Derivative : Derivative
  LOG_dPHI : Concatenate  NumInputs=1
  Mux : Mux  Inputs=2
  phidphi : Outport
  wires:
  phi/1 -> Mux/1, Derivative/1
  Mux/1 -> phidphi/1
  Derivative/1 -> LOG_dPHI/1
  LOG_dPHI/1 -> Mux/2

== system nmc/torque limiter ==
  torque : Inport
  Gain : Gain  Gain=0.01
  Gain1 : Gain  Gain=-1
  Product : Product
  Saturation : Saturate  UpperLimit=2  LowerLimit=0
  limited torque : Outport
  wires:
  Gain/1 -> Saturation/1
  [TorqueLimiterPercentage] -> Gain/1
  Product/1 -> limited torque/1
  torque/1 -> Product/2
  Gain1/1 -> Product/1
  Saturation/1 -> Gain1/1

== system nmc/torque limiter lopes ==
  torque : Inport
  Gain1 : Gain  Gain=0.01
  Product1 : Product
  Switch : Switch  Criteria=u2 > Threshold
  limited torque : Outport
  wires:
  Gain1/1 -> Product1/1
  [TorqueLimiterPercentage] -> Gain1/1
  torque/1 -> Product1/2, [NonLimitedOutput]
  [EnableTorqueLimiter] -> Switch/2
  Switch/1 -> limited torque/1
  Product1/1 -> [LimitedOutput]
  [LimitedOutput] -> Switch/1
  [NonLimitedOutput] -> Switch/3

== system nmc/AchillesNew/Left Side ==
  LphidphiAnkle : Inport
  AnkleJoint : nmc/NMC Joints/AnkleJoint
  SOL&TA Muscles : nmc/NMC Muscles/SOL&TA Muscles  VariableName=StimSOLL  VariableNameTA=StimTAL  SOLVM=SOLL_VM  TAVM=TAL_VM
  Selector7 : Selector  InputPortWidth=2  IndexOptions=Index vector (dialog)  Indices=[1 ]  OutputSizes=1
  Vector ConcatenateAnkle : Concatenate
  LTauAnkle : Outport
  wires:
  [LstanceOut] -> SOL&TA Muscles/2
  Selector7/1 -> SOL&TA Muscles/1
  [LTauAnkle] -> LTauAnkle/1
  LphidphiAnkle/1 -> [LphidphiAnkle]
  AnkleJoint/1 -> [LTauAnkle]
  [LphidphiAnkle] -> Selector7/1
  [LphidphiAnkle] -> AnkleJoint/1
  SOL&TA Muscles/1 -> Vector ConcatenateAnkle/1
  Vector ConcatenateAnkle/1 -> AnkleJoint/2
  SOL&TA Muscles/2 -> Vector ConcatenateAnkle/2

== system nmc/AchillesNew/Right Side ==
  RphidphiAnkle : Inport
  AnkleJoint : nmc/NMC Joints/AnkleJoint
  SOL&TA Muscles : nmc/NMC Muscles/SOL&TA Muscles  VariableName=StimSOLR  VariableNameTA=StimTAR  SOLVM=SOLL_VM  TAVM=TAL_VM
  Selector7 : Selector  InputPortWidth=2  IndexOptions=Index vector (dialog)  Indices=[1 ]  OutputSizes=1
  Vector ConcatenateAnkle : Concatenate
  RTauAnkle : Outport
  wires:
  [RTauAnkle] -> RTauAnkle/1
  RphidphiAnkle/1 -> [RphidphiAnkle]
  AnkleJoint/1 -> [RTauAnkle]
  [RstanceOut] -> SOL&TA Muscles/2
  [RphidphiAnkle] -> Selector7/1
  [RphidphiAnkle] -> AnkleJoint/1
  SOL&TA Muscles/1 -> Vector ConcatenateAnkle/1
  Vector ConcatenateAnkle/1 -> AnkleJoint/2
  Selector7/1 -> SOL&TA Muscles/1
  SOL&TA Muscles/2 -> Vector ConcatenateAnkle/2

== system nmc/AchillesNew_RealTime/Left Side ==
  LphidphiAnkle : Inport
  AnkleJoint : nmc/NMC Joints/AnkleJoint
  SOL&TA Muscles : nmc/NMC Muscles/SOL&TA Muscles  VariableName=StimSOLL  VariableNameTA=StimTAL  SOLVM=SOLL_VM  TAVM=TAL_VM
  Selector7 : Selector  InputPortWidth=2  IndexOptions=Index vector (dialog)  Indices=[1 ]  OutputSizes=1
  Vector ConcatenateAnkle : Concatenate
  LTauAnkle : Outport
  wires:
  SOL&TA Muscles/2 -> Vector ConcatenateAnkle/2
  Vector ConcatenateAnkle/1 -> AnkleJoint/2
  SOL&TA Muscles/1 -> Vector ConcatenateAnkle/1
  [LphidphiAnkle] -> AnkleJoint/1
  [LphidphiAnkle] -> Selector7/1
  AnkleJoint/1 -> [LTauAnkle]
  LphidphiAnkle/1 -> [LphidphiAnkle]
  [LTauAnkle] -> LTauAnkle/1
  Selector7/1 -> SOL&TA Muscles/1
  [LstanceOut] -> SOL&TA Muscles/2

== system nmc/AchillesNew_RealTime/Right Side ==
  RphidphiAnkle : Inport
  AnkleJoint : nmc/NMC Joints/AnkleJoint
  SOL&TA Muscles : nmc/NMC Muscles/SOL&TA Muscles  VariableName=StimSOLR  VariableNameTA=StimTAR  SOLVM=SOLL_VM  TAVM=TAL_VM
  Selector7 : Selector  InputPortWidth=2  IndexOptions=Index vector (dialog)  Indices=[1 ]  OutputSizes=1
  Vector ConcatenateAnkle : Concatenate
  RTauAnkle : Outport
  wires:
  SOL&TA Muscles/2 -> Vector ConcatenateAnkle/2
  Selector7/1 -> SOL&TA Muscles/1
  Vector ConcatenateAnkle/1 -> AnkleJoint/2
  SOL&TA Muscles/1 -> Vector ConcatenateAnkle/1
  [RphidphiAnkle] -> AnkleJoint/1
  [RphidphiAnkle] -> Selector7/1
  [RstanceOut] -> SOL&TA Muscles/2
  AnkleJoint/1 -> [RTauAnkle]
  RphidphiAnkle/1 -> [RphidphiAnkle]
  [RTauAnkle] -> RTauAnkle/1

== system nmc/AchillesOld_RealTime/Achilles ==
  AngleLeft : Inport
  IsStanceLeft : Inport  Port=2
  AngleRight : Inport  Port=3
  IsStanceRight : Inport  Port=4
  Add1 : Sum
  Add2 : Sum
  NMC_input_LeftAngle : Concatenate  NumInputs=1
  NMC_input_LeftStance : Concatenate  NumInputs=1
  NMC_input_RightAngle : Concatenate  NumInputs=1
  NMC_input_RightStance : Concatenate  NumInputs=1
  SOL&TA muscles left1 : nmc/NMC Muscles/SOL&TA Muscles  VariableName=StimSOLL  VariableNameTA=StimTAL  SOLVM=SOLL_VM  TAVM=TAL_VM
  SOL&TA muscles right : nmc/NMC Muscles/SOL&TA Muscles  VariableName=StimSOLR  VariableNameTA=StimTALR  SOLVM=SOLL_VM  TAVM=TAL_VM
  Torque : Outport
  Torque1 : Outport  Port=2
  wires:
  AngleLeft/1 -> NMC_input_LeftAngle/1
  NMC_input_LeftStance/1 -> SOL&TA muscles left1/2
  SOL&TA muscles left1/1 -> Add1/1
  SOL&TA muscles left1/2 -> Add1/2
  IsStanceLeft/1 -> NMC_input_LeftStance/1
  NMC_input_LeftAngle/1 -> SOL&TA muscles left1/1
  AngleRight/1 -> NMC_input_RightAngle/1
  NMC_input_RightStance/1 -> SOL&TA muscles right/2
  SOL&TA muscles right/1 -> Add2/1
  SOL&TA muscles right/2 -> Add2/2
  IsStanceRight/1 -> NMC_input_RightStance/1
  NMC_input_RightAngle/1 -> SOL&TA muscles right/1
  Add1/1 -> Torque/1
  Add2/1 -> Torque1/1

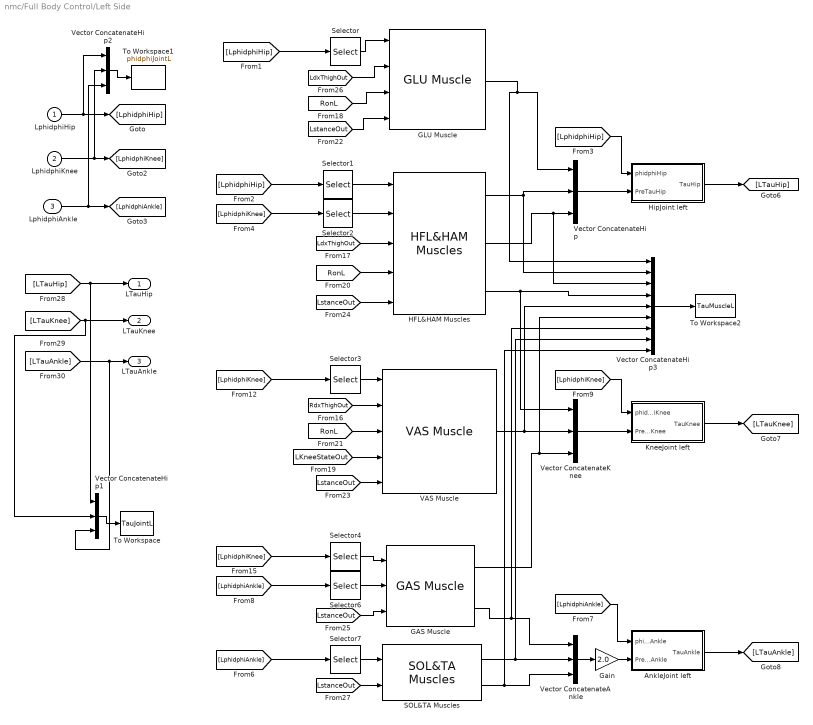
== system nmc/Full Body Control/Left Side ==
  LphidphiHip : Inport
  LphidphiKnee : Inport  Port=2
  LphidphiAnkle : Inport  Port=3
  AnkleJoint left : Subsystem
  GAS Muscle : nmc/NMC Muscles/GAS Muscle  VariableName=StimGASL  GASVM=GASL_VM
  GLU Muscle : nmc/NMC Muscles/GLU Muscle  StimGluSide=StimGLU1  GotoTag=GLUR_VM
  Gain : Gain  Gain=2.0
  HFL&HAM Muscles : nmc/NMC Muscles/HFL&HAM Muscles  StimHAMSide=StimHAM  StimHFLSide=StimHFL  HAMVM=HAMR_VM  HFLVM=HFLR_VM
  HipJoint left : Subsystem
  KneeJoint left : Subsystem
  SOL&TA Muscles : nmc/NMC Muscles/SOL&TA Muscles  VariableName=StimSOLL  VariableNameTA=StimTAL  SOLVM=SOLL_VM  TAVM=TAL_VM
  Selector{,1..4,6..7} (7 alike) : Selector  InputPortWidth=2  IndexOptions=Index vector (dialog)  Indices=[1 ]  OutputSizes=1
  To Workspace : ToWorkspace  VariableName=TauJointL  SaveFormat=Timeseries  SampleTime=-1
  To Workspace1 : ToWorkspace  VariableName=phidphiJointL  SaveFormat=Timeseries  SampleTime=-1
  To Workspace2 : ToWorkspace  VariableName=TauMuscleL  SaveFormat=Timeseries  SampleTime=-1
  VAS Muscle : nmc/NMC Muscles/VAS Muscle  VariableName=StimVAS  VASVM=VASR_VM
  Vector ConcatenateAnkle : Concatenate  NumInputs=3
  Vector ConcatenateHip : Concatenate  NumInputs=3
  Vector ConcatenateHip1 : Concatenate  NumInputs=3
  Vector ConcatenateHip2 : Concatenate  NumInputs=3
  Vector ConcatenateHip3 : Concatenate  NumInputs=9
  Vector ConcatenateKnee : Concatenate  NumInputs=3
  LTauHip : Outport
  LTauKnee : Outport  Port=2
  LTauAnkle : Outport  Port=3
  wires:
  Gain/1 -> AnkleJoint left/2(PreTauAnkle)
  GAS Muscle/2 -> Vector ConcatenateHip3/7, Vector ConcatenateAnkle/1
  Vector ConcatenateHip/1 -> HipJoint left/2(PreTauHip)
  [LphidphiKnee] -> KneeJoint left/1(phidphiKnee)
  Selector1/1 -> HFL&HAM Muscles/1
  Selector4/1 -> GAS Muscle/1
  [RdxThighOut] -> VAS Muscle/2
  SOL&TA Muscles/2 -> Vector ConcatenateHip3/9, Vector ConcatenateAnkle/3
  Vector ConcatenateAnkle/1 -> Gain/1
  Vector ConcatenateKnee/1 -> KneeJoint left/2(PreTauKnee)
  SOL&TA Muscles/1 -> Vector ConcatenateHip3/8, Vector ConcatenateAnkle/2
  Selector3/1 -> VAS Muscle/1
  Selector6/1 -> GAS Muscle/2
  VAS Muscle/1 -> Vector ConcatenateHip3/5, Vector ConcatenateKnee/2
  [LphidphiAnkle] -> AnkleJoint left/1(phidphiAnkle)
  GAS Muscle/1 -> Vector ConcatenateHip3/6, Vector ConcatenateKnee/3
  HFL&HAM Muscles/1 -> Vector ConcatenateHip/2, Vector ConcatenateHip3/2
  [LstanceOut] -> HFL&HAM Muscles/5
  [RonL] -> VAS Muscle/3
  [LphidphiKnee] -> Selector3/1
  [LphidphiKnee] -> Selector4/1
  [RonL] -> HFL&HAM Muscles/4
  [LKneeStateOut] -> VAS Muscle/4
  Selector/1 -> GLU Muscle/1
  [LstanceOut] -> GAS Muscle/3
  [LphidphiAnkle] -> Selector7/1
  HFL&HAM Muscles/2 -> Vector ConcatenateHip3/3, Vector ConcatenateHip/3
  Selector2/1 -> HFL&HAM Muscles/2
  [LphidphiAnkle] -> Selector6/1
  [LphidphiHip] -> Selector1/1
  [LstanceOut] -> VAS Muscle/5
  [LphidphiHip] -> Selector/1
  [LphidphiHip] -> HipJoint left/1(phidphiHip)
  [LphidphiKnee] -> Selector2/1
  HipJoint left/1(TauHip) -> [LTauHip]
  KneeJoint left/1(TauKnee) -> [LTauKnee]
  AnkleJoint left/1(TauAnkle) -> [LTauAnkle]
  [LdxThighOut] -> GLU Muscle/2
  [LstanceOut] -> GLU Muscle/4
  [RonL] -> GLU Muscle/3
  [LdxThighOut] -> HFL&HAM Muscles/3
  LphidphiHip/1 -> Vector ConcatenateHip2/1, [LphidphiHip]
  LphidphiKnee/1 -> Vector ConcatenateHip2/2, [LphidphiKnee]
  LphidphiAnkle/1 -> Vector ConcatenateHip2/3, [LphidphiAnkle]
  [LTauHip] -> Vector ConcatenateHip1/1, LTauHip/1
  [LTauAnkle] -> Vector ConcatenateHip1/3, LTauAnkle/1
  Vector ConcatenateHip1/1 -> To Workspace/1
  Vector ConcatenateHip2/1 -> To Workspace1/1
  [LTauKnee] -> LTauKnee/1, Vector ConcatenateHip1/2
  Vector ConcatenateHip3/1 -> To Workspace2/1
  GLU Muscle/1 -> Vector ConcatenateHip3/1, Vector ConcatenateHip/1
  Selector7/1 -> SOL&TA Muscles/1
  [LstanceOut] -> SOL&TA Muscles/2
  HFL&HAM Muscles/3 -> Vector ConcatenateKnee/1, Vector ConcatenateHip3/4

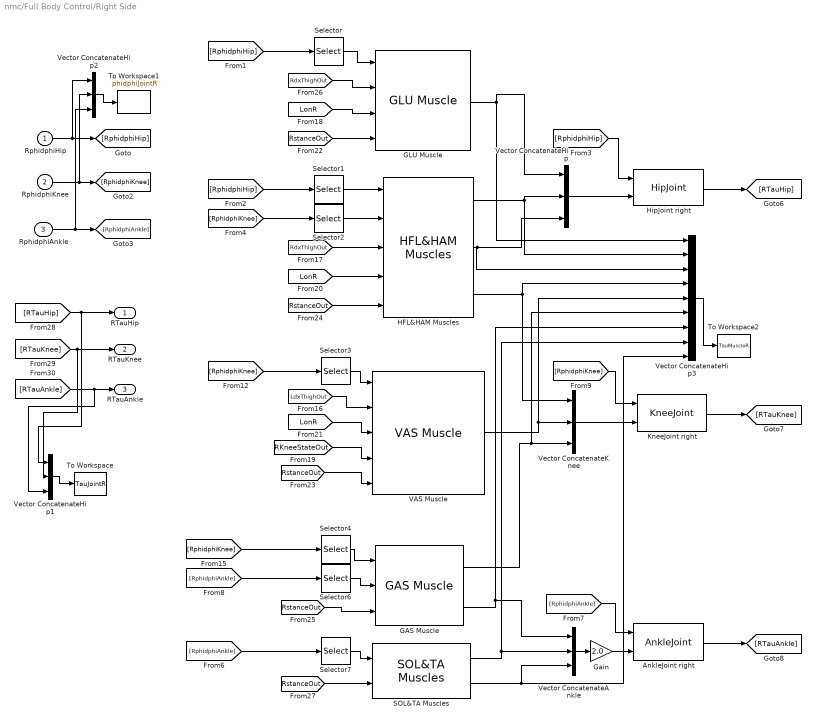
== system nmc/Full Body Control/Right Side ==
  RphidphiHip : Inport
  RphidphiKnee : Inport  Port=2
  RphidphiAnkle : Inport  Port=3
  AnkleJoint right : nmc/NMC Joints/AnkleJoint
  GAS Muscle : nmc/NMC Muscles/GAS Muscle  VariableName=StimGASR  GASVM=GASL_VM
  GLU Muscle : nmc/NMC Muscles/GLU Muscle  StimGluSide=StimGLUR  GotoTag=GLUR_VM
  Gain : Gain  Gain=2.0
  HFL&HAM Muscles : nmc/NMC Muscles/HFL&HAM Muscles  StimHAMSide=StimHAMR  StimHFLSide=StimHFLR  HAMVM=HAMR_VM  HFLVM=HFLR_VM
  HipJoint right : nmc/NMC Joints/HipJoint
  KneeJoint right : nmc/NMC Joints/KneeJoint
  SOL&TA Muscles : nmc/NMC Muscles/SOL&TA Muscles  VariableName=StimSOLR  VariableNameTA=StimTAR  SOLVM=SOLL_VM  TAVM=TAL_VM
  Selector{,1..4,6..7} (7 alike) : Selector  InputPortWidth=2  IndexOptions=Index vector (dialog)  Indices=[1 ]  OutputSizes=1
  To Workspace : ToWorkspace  VariableName=TauJointR  SaveFormat=Timeseries  SampleTime=-1
  To Workspace1 : ToWorkspace  VariableName=phidphiJointR  SaveFormat=Timeseries  SampleTime=-1
  To Workspace2 : ToWorkspace  VariableName=TauMuscleR  SaveFormat=Timeseries  SampleTime=-1
  VAS Muscle : nmc/NMC Muscles/VAS Muscle  VariableName=StimVASR  VASVM=VASR_VM
  Vector ConcatenateAnkle : Concatenate  NumInputs=3
  Vector ConcatenateHip : Concatenate  NumInputs=3
  Vector ConcatenateHip1 : Concatenate  NumInputs=3
  Vector ConcatenateHip2 : Concatenate  NumInputs=3
  Vector ConcatenateHip3 : Concatenate  NumInputs=9
  Vector ConcatenateKnee : Concatenate  NumInputs=3
  RTauHip : Outport
  RTauKnee : Outport  Port=2
  RTauAnkle : Outport  Port=3
  wires:
  Gain/1 -> AnkleJoint right/2
  GAS Muscle/2 -> Vector ConcatenateHip3/7, Vector ConcatenateAnkle/1
  Vector ConcatenateHip/1 -> HipJoint right/2
  [RphidphiKnee] -> KneeJoint right/1
  Selector1/1 -> HFL&HAM Muscles/1
  Selector4/1 -> GAS Muscle/1
  [LdxThighOut] -> VAS Muscle/2
  SOL&TA Muscles/2 -> Vector ConcatenateAnkle/3, Vector ConcatenateHip3/9
  Selector7/1 -> SOL&TA Muscles/1
  Vector ConcatenateAnkle/1 -> Gain/1
  Vector ConcatenateKnee/1 -> KneeJoint right/2
  SOL&TA Muscles/1 -> Vector ConcatenateHip3/8, Vector ConcatenateAnkle/2
  Selector3/1 -> VAS Muscle/1
  Selector6/1 -> GAS Muscle/2
  VAS Muscle/1 -> Vector ConcatenateHip3/5, Vector ConcatenateKnee/2
  [RphidphiAnkle] -> AnkleJoint right/1
  GAS Muscle/1 -> Vector ConcatenateHip3/6, Vector ConcatenateKnee/3
  HFL&HAM Muscles/1 -> Vector ConcatenateHip3/2, Vector ConcatenateHip/2
  GLU Muscle/1 -> Vector ConcatenateHip3/1, Vector ConcatenateHip/1
  [LonR] -> VAS Muscle/3
  [RphidphiKnee] -> Selector3/1
  [RphidphiKnee] -> Selector4/1
  [RKneeStateOut] -> VAS Muscle/4
  HFL&HAM Muscles/3 -> Vector ConcatenateKnee/1, Vector ConcatenateHip3/4
  Selector/1 -> GLU Muscle/1
  [RstanceOut] -> GAS Muscle/3
  [RphidphiAnkle] -> Selector7/1
  [RstanceOut] -> SOL&TA Muscles/2
  HFL&HAM Muscles/2 -> Vector ConcatenateHip3/3, Vector ConcatenateHip/3
  Selector2/1 -> HFL&HAM Muscles/2
  [RphidphiAnkle] -> Selector6/1
  [RphidphiHip] -> Selector1/1
  [RstanceOut] -> VAS Muscle/5
  [RphidphiHip] -> Selector/1
  [RphidphiHip] -> HipJoint right/1
  [RphidphiKnee] -> Selector2/1
  HipJoint right/1 -> [RTauHip]
  KneeJoint right/1 -> [RTauKnee]
  AnkleJoint right/1 -> [RTauAnkle]
  [RdxThighOut] -> GLU Muscle/2
  [LonR] -> GLU Muscle/3
  [RstanceOut] -> GLU Muscle/4
  [RdxThighOut] -> HFL&HAM Muscles/3
  [LonR] -> HFL&HAM Muscles/4
  [RstanceOut] -> HFL&HAM Muscles/5
  RphidphiHip/1 -> Vector ConcatenateHip2/1, [RphidphiHip]
  RphidphiKnee/1 -> Vector ConcatenateHip2/2, [RphidphiKnee]
  RphidphiAnkle/1 -> [RphidphiAnkle], Vector ConcatenateHip2/3
  [RTauHip] -> Vector ConcatenateHip1/1, RTauHip/1
  [RTauKnee] -> Vector ConcatenateHip1/2, RTauKnee/1
  [RTauAnkle] -> Vector ConcatenateHip1/3, RTauAnkle/1
  Vector ConcatenateHip1/1 -> To Workspace/1
  Vector ConcatenateHip2/1 -> To Workspace1/1
  Vector ConcatenateHip3/1 -> To Workspace2/1

== system nmc/Full Body Control/Sensors ==
  Theta : Inport
  dTheta : Inport  Port=2
  LdxThigh : Inport  Port=3
  RdxThigh : Inport  Port=4
  LKneeState : Inport  Port=5
  RKneeState : Inport  Port=6
  LStance : Inport  Port=7
  RStance : Inport  Port=8
  FootSensor : nmc/FootSensor
  KneeSensor : nmc/KneeSensor
  ThightSensor : nmc/ThightSensor
  UpperBodyOrientation : nmc/UpperBodyOrientation
  tag scope: LKneeStateOut=global, LdxThighOut=global, LonR=global, LstanceOut=global, RKneeStateOut=global, RdxThighOut=global, RonL=global, RstanceOut=global
  wires:
  RStance/1 -> FootSensor/2
  LStance/1 -> FootSensor/1
  RKneeState/1 -> KneeSensor/2
  LKneeState/1 -> KneeSensor/1
  RdxThigh/1 -> ThightSensor/2
  LdxThigh/1 -> ThightSensor/1
  dTheta/1 -> UpperBodyOrientation/2
  Theta/1 -> UpperBodyOrientation/1
  FootSensor/4 -> [RonL]
  FootSensor/3 -> [LonR]
  FootSensor/2 -> [RstanceOut]
  FootSensor/1 -> [LstanceOut]
  KneeSensor/2 -> [RKneeStateOut]
  KneeSensor/1 -> [LKneeStateOut]
  ThightSensor/1 -> [LdxThighOut]
  ThightSensor/2 -> [RdxThighOut]

== system nmc/LeftSwing/CPG ==
  freq : Inport
  Enable : EnablePort
  LoadFromWorkspace : FromWorkspace  VariableName=CPG.Signals.NominalShape1.Value  SampleTime=0
  MorphOscillator : nmc/MorphOscillator
  y : Outport
  wires:
  MorphOscillator/1 -> y/1
  freq/1 -> MorphOscillator/2
  LoadFromWorkspace/1 -> MorphOscillator/1

== system nmc/LeftSwing/GenerateAndSaveNominalShape ==
  switch_signal : Inport
  signal : Inport  Port=2
  swingOrstance : Inport  Port=3
  Enable : EnablePort
  NominalShapeGenerator : nmc/Save  SystemSampleTime=-1
  SaveToWorkspace : Subsystem
  wires:
  switch_signal/1 -> NominalShapeGenerator/1
  signal/1 -> NominalShapeGenerator/2
  swingOrstance/1 -> NominalShapeGenerator/3
  NominalShapeGenerator/2 -> SaveToWorkspace/1(In1)
  NominalShapeGenerator/1 -> SaveToWorkspace/Enable

== system nmc/LeftSwing/LeftOrRight ==
  side : Inport
  Switch : Switch  Criteria=u2 > Threshold
  switch_signal : Outport
  wires:
  [CPG_leftSwitchSignal] -> Switch/1
  side/1 -> Switch/2
  Switch/1 -> switch_signal/1
  [CPG_rightSwitchSignal] -> Switch/3

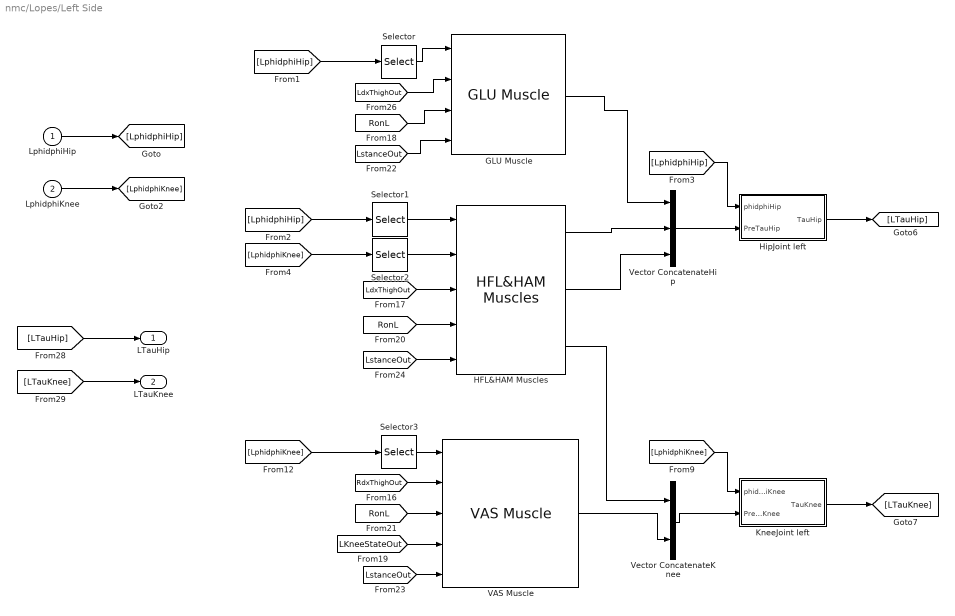
== system nmc/Lopes/Left Side ==
  LphidphiHip : Inport
  LphidphiKnee : Inport  Port=2
  GLU Muscle : nmc/NMC Muscles/GLU Muscle  StimGluSide=StimGLU1  GotoTag=GLUR_VM
  HFL&HAM Muscles : nmc/NMC Muscles/HFL&HAM Muscles  StimHAMSide=StimHAM  StimHFLSide=StimHFL  HAMVM=HAMR_VM  HFLVM=HFLR_VM
  HipJoint left : Subsystem
  KneeJoint left : Subsystem
  Selector{,1..3} (4 alike) : Selector  InputPortWidth=2  IndexOptions=Index vector (dialog)  Indices=[1 ]  OutputSizes=1
  VAS Muscle : nmc/NMC Muscles/VAS Muscle  VariableName=StimVAS  VASVM=VASR_VM
  Vector ConcatenateHip : Concatenate  NumInputs=3
  Vector ConcatenateKnee : Concatenate
  LTauHip : Outport
  LTauKnee : Outport  Port=2
  wires:
  Vector ConcatenateHip/1 -> HipJoint left/2(PreTauHip)
  [LphidphiKnee] -> KneeJoint left/1(phidphiKnee)
  Selector1/1 -> HFL&HAM Muscles/1
  [RdxThighOut] -> VAS Muscle/2
  Vector ConcatenateKnee/1 -> KneeJoint left/2(PreTauKnee)
  Selector3/1 -> VAS Muscle/1
  VAS Muscle/1 -> Vector ConcatenateKnee/2
  HFL&HAM Muscles/1 -> Vector ConcatenateHip/2
  [LstanceOut] -> HFL&HAM Muscles/5
  [RonL] -> VAS Muscle/3
  [LphidphiKnee] -> Selector3/1
  [RonL] -> HFL&HAM Muscles/4
  [LKneeStateOut] -> VAS Muscle/4
  Selector/1 -> GLU Muscle/1
  HFL&HAM Muscles/2 -> Vector ConcatenateHip/3
  Selector2/1 -> HFL&HAM Muscles/2
  [LphidphiHip] -> Selector1/1
  [LstanceOut] -> VAS Muscle/5
  [LphidphiHip] -> Selector/1
  [LphidphiHip] -> HipJoint left/1(phidphiHip)
  [LphidphiKnee] -> Selector2/1
  HipJoint left/1(TauHip) -> [LTauHip]
  KneeJoint left/1(TauKnee) -> [LTauKnee]
  [LdxThighOut] -> GLU Muscle/2
  [LstanceOut] -> GLU Muscle/4
  [RonL] -> GLU Muscle/3
  [LdxThighOut] -> HFL&HAM Muscles/3
  LphidphiHip/1 -> [LphidphiHip]
  LphidphiKnee/1 -> [LphidphiKnee]
  [LTauHip] -> LTauHip/1
  [LTauKnee] -> LTauKnee/1
  GLU Muscle/1 -> Vector ConcatenateHip/1
  HFL&HAM Muscles/3 -> Vector ConcatenateKnee/1
